simulink library "LLA2ECEF"  (R2018b)
settings: Solver=VariableStepAuto  StartTime=0.0  StopTime=10.0  RelTol=1e-3
settings Model: Creator=BI28030  LastModifiedBy=BI28030

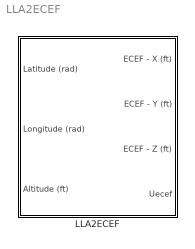
== system LLA2ECEF ==
  LLA2ECEF : Subsystem  mask(LLA2ECEF){a=6378137, b=6356752.31424518}
      mask prompts: a "Semi-major axis (meters)"; b "Semi-minor axis (meters)"
      mask help:
      | Calculates the equivalent Earth-Centered Earth-Fixed coordinates for a
      | given location expressed in geodetic Latitude, Longitude and Altitude.
      |
      | Also produces matrix that can rotate East-North-Up velocity
      | into ECEF velocity
      mask Help:
      | Calculates the equivalent Earth-Centered Earth-Fixed coordinates for a
      | given location expressed in geodetic Latitude, Longitude and Altitude.
      | 
      | Also produces matrix that can rotate East-North-Up velocity
      | into ECEF velocity

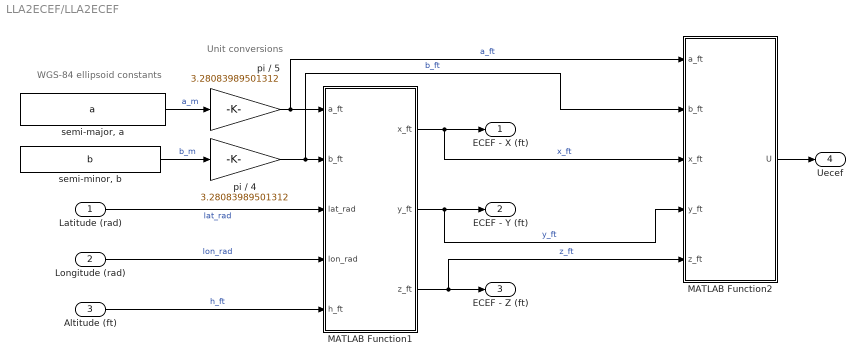
== system LLA2ECEF/LLA2ECEF ==
  note: Unit conversions
  note: WGS-84 ellipsoid constants
  Latitude (rad) : Inport
  Longitude (rad) : Inport  Port=2
  Altitude (ft) : Inport  Port=3
  MATLAB Function1 : MATLAB Function  TreatAsAtomicUnit=on
  MATLAB Function2 : MATLAB Function  TreatAsAtomicUnit=on
  pi / 4 : Gain  Gain=3.28083989501312
  pi / 5 : Gain  Gain=3.28083989501312
  "semi-major, a" : Constant  Value=a
  "semi-minor, b" : Constant  Value=b
  ECEF - X (ft) : Outport
  ECEF - Y (ft) : Outport  Port=2
  ECEF - Z (ft) : Outport  Port=3
  Uecef : Outport  Port=4  OutDataTypeStr=double  PortDimensions=[3 3]
  wires:
  pi / 4/1 -> MATLAB Function2/2(b_ft), MATLAB Function1/2(b_ft)  "b_ft"
  pi / 5/1 -> MATLAB Function2/1(a_ft), MATLAB Function1/1(a_ft)  "a_ft"
  MATLAB Function1/1(x_ft) -> MATLAB Function2/3(x_ft), ECEF - X (ft)/1  "x_ft"
  MATLAB Function1/2(y_ft) -> MATLAB Function2/4(y_ft), ECEF - Y (ft)/1  "y_ft"
  MATLAB Function1/3(z_ft) -> MATLAB Function2/5(z_ft), ECEF - Z (ft)/1  "z_ft"
  Altitude (ft)/1 -> MATLAB Function1/5(h_ft)  "h_ft"
  Longitude (rad)/1 -> MATLAB Function1/4(lon_rad)  "lon_rad"
  Latitude (rad)/1 -> MATLAB Function1/3(lat_rad)  "lat_rad"
  "semi-major, a"/1 -> pi / 5/1  "a_m"
  "semi-minor, b"/1 -> pi / 4/1  "b_m"
  MATLAB Function2/1(U) -> Uecef/1

== matlab function LLA2ECEF/MATLAB Function2 ==
  data: a_ft input; b_ft input; x_ft input; y_ft input; z_ft input; U output
function U = ECEFRotMat(a_ft,b_ft,x_ft,y_ft,z_ft)
% Produce matrix U = [ Ehat_ECEF Nhat_ECEF Uhat_ECEF ]

f = (a_ft-b_ft)/a_ft; % flattening

posECEF0 = [ x_ft y_ft z_ft ];

    % Compute the local Up unit vector
    vHatU = posECEF0';
    vHatU(3) = vHatU(3) ./ ((1-f)^2);
    vHatU = vHatU ./ norm(vHatU);

    % Compute the projection onto the local Up vector
    pU = vHatU * vHatU';

    % Compute the projection onto the local Tangent plane
    pT = eye(3) - pU;

    % Compute the local North unit vector
    vHatZ = [0;0;1];
    vHatN = pT * vHatZ;
    vHatN = vHatN ./ norm(vHatN);

    % Compute the local East unit vector
    vHatE = cross(vHatN,vHatU);

    % Compute ENU rotation matrix
    U = [ vHatE vHatN vHatU ];

== matlab function LLA2ECEF/MATLAB Function1 ==
  data: x_ft output; a_ft input; y_ft output; b_ft input; lat_rad input; lon_rad input; h_ft input; z_ft output
function [x_ft,y_ft,z_ft] = LLA2ECEF(a_ft,b_ft,lat_rad,lon_rad,h_ft)
%#codegen

% First eccentricity
e = sqrt((a_ft^2-b_ft^2)/a_ft^2); 

% Ellipsoidal "radius"
N = a_ft./sqrt(1-(e^2).*sin(lat_rad).^2);

% ECEF coordinates (meters)
x_ft = (N + h_ft)*cos(lat_rad)*cos(lon_rad);
y_ft = (N + h_ft)*cos(lat_rad)*sin(lon_rad);
z_ft = (((b_ft^2)/(a_ft^2))*N + h_ft)*sin(lat_rad);
